simulink model "thermostatController_SimHarness"  (R2023a)
settings: Solver=VariableStepAuto  StartTime=0.0  StopTime=30  MaxStep=0.01  RelTol=1e-4  EnableMultiTasking=on
PreLoadFcn:
  | thermal_data
  | setupPID
InitFcn:
  | thermal_data
  | setupPID
model workspace (MAT data in the model file):
  desired_temp = 30
undefined symbols (not defined in the file): c, M, Mdot, Req, TinIC
settings Model: Creator=llemke  LastModifiedBy=Sam
settings SolverCC: AlgebraicLoopSolver=TrustRegion
settings DataIOCC: LimitDataPoints=on  SaveOutput=off  SaveTime=off
settings OptimizationCC: ExpressionDepthLimit=2147483647  LifeSpan=1
settings DebuggingCC: UnderspecifiedInitializationDetection=Classic  MergeDetectMultiDrivingBlocksExec=none  FcnCallInpInsideContextMsg=warning  UnconnectedInputMsg=warning  UnconnectedOutputMsg=warning  UnconnectedLineMsg=warning  AllowSymbolicDim=off  StateNameClashWarn=warning  SFUnexpectedBacktrackingDiag=warning  SFNoUnconditionalDefaultTransitionDiag=warning  SFExecutionAtInitializationDiag=none  ArithmeticOperatorsInVariantConditions=warning
settings ModelReferenceCC: EnableRefExpFcnMdlSchedulingChecks=on
settings SFSimCC: SimUseLocalCustomCode=off  CustomCodeUndefinedFunction=UseInterfaceOnly
settings RTWCC: RTWUseLocalCustomCode=off  DLArmComputeVersion=19.05
settings CodeAppCC: StateflowObjectComments=on
settings GRTTargetCC: TargetLangStandard=C89/C90 (ANSI)  CombineOutputUpdateFcns=off  GRTInterface=on

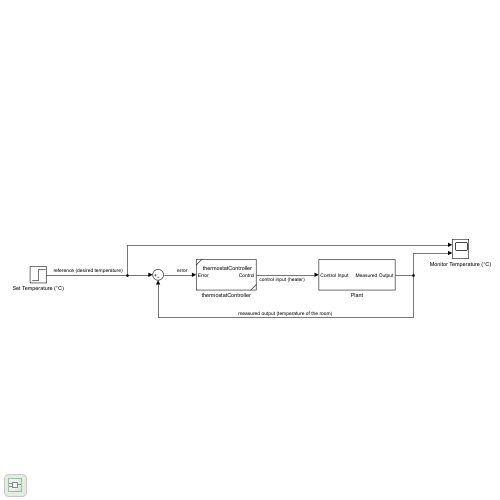
[thumbnail: Simulink's stored preview of the top-level diagram]
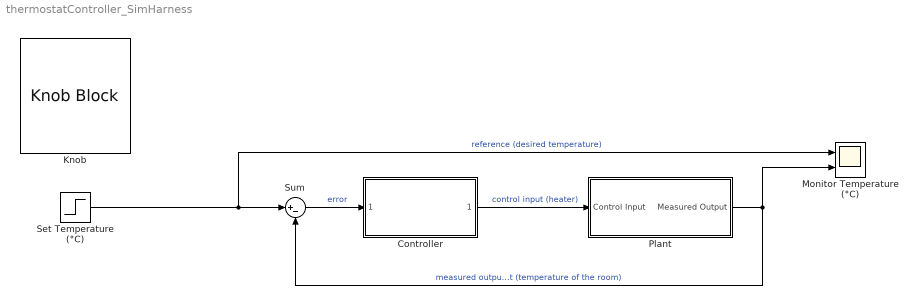
== system thermostatController_SimHarness ==
  Controller : Subsystem  ReferencedSubsystem=thermostatController
  Knob : KnobBlock
  Monitor Temperature (°C) : Scope  NumInputPorts=2
  Plant : Subsystem
  Set Temperature (°C) : Step  Time=5  After=30  SampleTime=0
  Sum : Sum  Inputs=|+-
  wires:
  Set Temperature (°C)/1 -> Sum/1, Monitor Temperature (°C)/1  "reference (desired temperature)"
  Plant/1(Measured Output) -> Monitor Temperature (°C)/2, Sum/2  "measured output (temperature of the room)"
  Sum/1 -> Controller/1  "error"
  Controller/1 -> Plant/1(Control Input)  "control input (heater)"

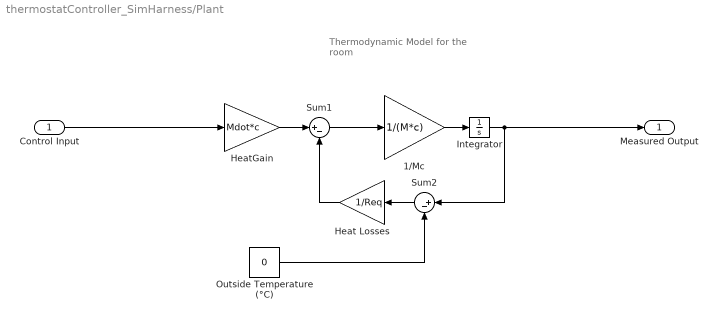
== system thermostatController_SimHarness/Plant ==
  note: Thermodynamic Model
      | for the room
  Control Input : Inport
  1/Mc : Gain  Gain=1/(M*c)  SaturateOnIntegerOverflow=on  OutDataTypeStr=Inherit: Same as input  ParamDataTypeStr=Inherit: Same as input
  Heat Losses : Gain  Gain=1/Req  SaturateOnIntegerOverflow=on  OutDataTypeStr=Inherit: Same as input  ParamDataTypeStr=Inherit: Same as input
  HeatGain : Gain  Gain=Mdot*c
  Integrator : Integrator  InitialCondition=TinIC
  Outside Temperature (°C) : Constant  Value=0
  Sum1 : Sum  Inputs=|+-  InputSameDT=on  SaturateOnIntegerOverflow=on  OutDataTypeStr=Inherit: Same as first input
  Sum2 : Sum  Inputs=|+-  InputSameDT=on  SaturateOnIntegerOverflow=on  OutDataTypeStr=Inherit: Same as first input
  Measured Output : Outport
  wires:
  Control Input/1 -> HeatGain/1
  Sum1/1 -> 1/Mc/1
  Outside Temperature (°C)/1 -> Sum2/2
  Integrator/1 -> Measured Output/1, Sum2/1
  Sum2/1 -> Heat Losses/1
  1/Mc/1 -> Integrator/1
  Heat Losses/1 -> Sum1/2
  HeatGain/1 -> Sum1/1
